simulink model "PubIfDecisionTOS_MDL"  (R2020b)
settings: configuration reference "DspaceConfig" (kept outside this file)
PostLoadFcn:
  | if any(exist('dsrtsu_mdlpostloadfcn', 'file') ~= 0), dsrtsu_mdlpostloadfcn('Execute', bdroot); end
InitFcn:
  | , if any(exist('dsmpb_private', 'file') ~= 0), dsmpb_private('dsmpb_mdlclblib', 'Init', bdroot); end,
undefined symbols (not defined in the file or in its folder): C_TOS_ACCEgoRAxletoFbumplength_m, C_TOS_ACCTargetFront_Flag, C_TOS_AEBJAPedObjDxThre_Val, C_TOS_AEBJAPedObjDyThre_Val, C_TOS_AEBJATargetSize_Val, C_TOS_AEBJAVehObjDxThre_Val, C_TOS_AEBJAVehObjDyThre_Val, C_TOS_AEBJuncPedTargetSize_Val, C_TOS_AEBLatObjDxThre_Val, C_TOS_AEBLatPedDyThre_Val, C_TOS_AEBLatTargetSize_Val, C_TOS_AEBLongTargetInEgoFront_Flag, C_TOS_axAbsGround_Parameter, C_TOS_CameraConfirmedFlag, C_TOS_CNsubjWidth, C_TOS_CurrentLaneCoreMinWidth_Val, C_TOS_CutInProb_Val_Zero, C_TOS_CutOutProb_Val_Zero, C_TOS_D2R_Val, C_TOS_DefaultValueObjectToCenterLine_dy, C_TOS_EgoCarWidth_Val, C_TOS_EgoDxRefPoint_m, C_TOS_EgoRAxletoFbumplength_m, C_TOS_HalfWidthVehicle_Con, C_TOS_HWA_CurrentLaneFlag, C_TOS_HWA_LeftLaneFlag, C_TOS_HWA_MovingDir_Vaild, C_TOS_HWA_MovState_Vaild, C_TOS_HWA_RightLaneFlag, C_TOS_LaneLineCourseErrorFront, C_TOS_LaneLineCourseErrorRear, C_TOS_MotorbikeDefaultWidth_m, C_TOS_NumberOfEffectiveTargets, C_TOS_Obj_Age_Val, C_TOS_Objdx_Constraint_Val, C_TOS_ObjectDefaultWidth_m, C_TOS_ObjInCurrentLane_Val, C_TOS_ObjInCurrentLaneValid, C_TOS_ObjInLeftLaneValid, C_TOS_ObjInRightLaneValid, C_TOS_ObjNotInCurrentLane_Val, C_TOS_ObjNotREElementType, C_TOS_ObjPredictDis_dy_ConstantVal_Zeros, C_TOS_ObjToCenterLine_ConstantVal_Zeros, C_TOS_OFMObjIDInvilad_Val, C_TOS_PIL_LatDisCons_Val_zero, C_TOS_PIL_ObjectCutInFlag_b, C_TOS_PIL_ObjectCutOutFlag_b, C_TOS_PIL_ObjLaneProb_al_Val, C_TOS_PP_ObjFusType_FC_Confirm_b, C_TOS_PP_ObjFusType_FC_FR_Confirm_b, C_TOS_PP_ObjFusType_FR_Confirm_b, C_TOS_RE_80BoolDefault_Val, C_TOS_RE_80Single181Default_Val, C_TOS_RE_80Single255Default_Val, C_TOS_RE_80Uint8Default_Val, C_TOS_RE_D2R, C_TOS_RE_D_180_Val, C_TOS_RE_InvalidObjectID_Val, C_TOS_RE_InvalidTargetChainDir_Val ... (+142)
libraries: simulink x1650, TOS_LIB x361, canfdmsglib x14
(part 62 of 69)

== stateflow chart PubIfDecisionTOS_MDL/TOS_20201112/TOS_2012080320/PIL_1029/OverlapRatio_Calculate/PIL_OverlapCalculation/OverlapRatioCalcFlow ==
  state overlapRatio = overlapRatioCalc(dyCriticalEgoObj,dyOverlapActual) [function]
  (default) -> (junction 33)
  (junction 33) -> (junction 2) : {
      | 	dyOverlapActual = dyEgo2Center - dyObject2Center;
      |
      | }
  (junction 2) -> (junction 3) [order 1] : [dyOverlapActual == 0]
  (junction 2) -> (junction 7) [order 2] : {
      | 	dyOverlapActualAbs = abs(dyOverlapActual);
      | }
  (junction 3) -> (junction 5) : {
      | 	tempOverlapRatio = 1;
      | }
  (junction 7) -> (junction 9) [order 1] : [dyOverlapActualAbs > dyCriticalEgoObj ]
  (junction 7) -> (junction 13) [order 2] : {
      | 	tempOverlapRatio = overlapRatioCalc(dyCriticalEgoObj,dyOverlapActual);
      | }
  (junction 9) -> (junction 11) : {
      | 	tempOverlapRatio = 0;
      | }
  (junction 11) -> (junction 13)
  (junction 5) -> (junction 11)
  (junction 13) -> (junction 17) : {
      | 	overlapRatio = tempOverlapRatio;
      | }
  data: dyCriticalEgoObj function_input; dyOverlapActual function_input; overlapRatio function_output; dyCriticalEgoObj input; dyEgo2Center input; overlapRatio output; tempOverlapRatio local double; dyOverlapActualAbs local double; dyObject2Center input; dyOverlapActual local double

== matlab function PubIfDecisionTOS_MDL/TOS_20201112/TOS_2012080320/PIL_1029/PIL_ObjectToCenterLine_dy_Filt/PIL_ObjectToCenterLine_dy/Subsystem/ObjectToCenterLine_dyFilit ==
  data: ObjectID_Filt_K1 input uint8; ObjectToCenterLine_dy_Filt_K1 input single; ObjectToCenterLine_dy input single; ObjectToCenterLine_dy_Filt output single; Object_ID input uint8; TOS_OFMObjValid_Flag input; P_TOS_PIL_ObjectToCenterLine_dy_CutInUpperLimit input single; P_TOS_PIL_ObjectToCenterLine_dy_CutInDeclineLimit input; Iterator_Num input int32
function ObjectToCenterLine_dy_Filt = fcn(ObjectID_Filt_K1,ObjectToCenterLine_dy_Filt_K1,ObjectToCenterLine_dy,...
    Object_ID,TOS_OFMObjValid_Flag,P_TOS_PIL_ObjectToCenterLine_dy_CutInUpperLimit,P_TOS_PIL_ObjectToCenterLine_dy_CutInDeclineLimit, Iterator_Num)

% Iterator_Num = uint8(80);
% K_FiltingParmet_RightLanepil=single(0);
ObjectToCenterLine_dy_Filt = single(0);


if  Object_ID ~=uint8(0) && TOS_OFMObjValid_Flag~=uint8(0)
        for  i=1: int32(Iterator_Num)
            if   ObjectID_Filt_K1(i) == Object_ID && ObjectID_Filt_K1(i)~=uint8(0)  && Object_ID~=uint8(0)   % 目标当前Object_ID 与历史值ObjectID_Filt_K1相同时；滤波处理

                    if ObjectToCenterLine_dy > ObjectToCenterLine_dy_Filt_K1(i) 
                          ObjectToCenterLine_dy_Filt = ObjectToCenterLine_dy_Filt_K1(i) + ...
                          P_TOS_PIL_ObjectToCenterLine_dy_CutInUpperLimit*( ObjectToCenterLine_dy - ObjectToCenterLine_dy_Filt_K1(i)); 
                    else
                         ObjectToCenterLine_dy_Filt = ObjectToCenterLine_dy_Filt_K1(i) + ...
                          P_TOS_PIL_ObjectToCenterLine_dy_CutInDeclineLimit*( ObjectToCenterLine_dy - ObjectToCenterLine_dy_Filt_K1(i)); 
                    end

                    break;
            else
                if i==Iterator_Num    % 如果当前Object_ID首次出现；输出当前值为ObjectToCenterLine_dy_Filt
                    ObjectToCenterLine_dy_Filt = ObjectToCenterLine_dy;        
                else
                    ObjectToCenterLine_dy_Filt = ObjectToCenterLine_dy;  
                end
            end 
        end
else
      ObjectToCenterLine_dy_Filt = ObjectToCenterLine_dy;  
end

== matlab function PubIfDecisionTOS_MDL/TOS_20201112/TOS_2012080320/PP1128/AAT-AdditionalAttributes/PP_ObjFirstDxDyDetermineSignalProcessing/PP_ObjFirstDxDyDetermine/PP_ObjFirstDxDyDetermine/MATLAB Function ==
  data: Object_ID input; Obj_DxFD output; Object_Dx input; Object_Dy input; Object_ID_Last input; Object_Dx_Last input; Object_Dy_Last input; Obj_DyFD output; C_NumberOfEffectiveTargets input
function [Obj_DxFD,Obj_DyFD] = fcn(Object_ID,Object_Dx,Object_Dy,Object_ID_Last,Object_Dx_Last,Object_Dy_Last,C_NumberOfEffectiveTargets)
objindex=uint8(0);
for i=1:C_NumberOfEffectiveTargets
    if Object_ID_Last(i)==Object_ID && Object_ID_Last(i)~=uint8(0)
        objindex=uint8(i);
        break
    end
end
if objindex~=0
    Obj_DxFD=single(Object_Dx_Last(objindex));
    Obj_DyFD=single(Object_Dy_Last(objindex));
else
    Obj_DxFD=single(Object_Dx);
    Obj_DyFD=single(Object_Dy);
end

== matlab function PubIfDecisionTOS_MDL/TOS_20201112/TOS_2012080320/PP1128/AAT-AdditionalAttributes/PP_ObjectToCenterLine_dy/PP_ObjectToCenterLine_vyc/ObjVyc ==
  data: ObjVyc output single; Line04_PC2 input single size=1; Line04_PC1 input single size=1; Line04_dDisStart input single size=1; Line04_dDisEnd input single size=1; Line05_PC2 input single size=1; Line05_PC1 input single size=1; Line05_dDisStart input single size=1; Line05_dDisEnd input single size=1; Line06_PC2 input single size=1; Line06_PC1 input single size=1; Line06_dDisStart input single size=1; Line06_dDisEnd input single size=1; Obj_ID input uint8 size=80; Obj_Dx input single size=80; Obj_VxG input single size=80; Obj_VyG input single size=80; TOS_OFMObjValid_Flag input uint8; vxvRefMs input; C_NumberOfEffectiveTargets input int32 size=1
function ObjVyc  = ObjVyc( Line04_PC2,Line04_PC1,Line04_dDisStart,Line04_dDisEnd,...
                           Line05_PC2,Line05_PC1,Line05_dDisStart,Line05_dDisEnd,...
                           Line06_PC2,Line06_PC1,Line06_dDisStart,Line06_dDisEnd,...
                           Obj_ID,Obj_Dx,Obj_VxG,Obj_VyG,TOS_OFMObjValid_Flag, vxvRefMs,C_NumberOfEffectiveTargets)

 Iterator_Num = int32(80);                      
                       
ObjVyc = single(zeros(Iterator_Num,1));

for i=int32(1):int32(C_NumberOfEffectiveTargets)
    if Obj_ID(i) ~= uint8(0) && TOS_OFMObjValid_Flag(i) ~= uint8(0)
       t_dxv = Obj_Dx(i);  %车体系X方向距离，目标到后轴中心距离
       t_VxG = vxvRefMs+Obj_VxG(i); %车体系目标X方向绝对速度
       t_VyG = Obj_VyG(i); %车体系y方向绝对速度（自车VY=0）
%---------------------------------------------------------------------------------------------------------------------     
       t_bParabolaYNLane = single(1);
       t_bParabolaXNLane = single(1);  
       
       if t_dxv > Line04_dDisStart && t_dxv < Line04_dDisEnd
           temp1 =  single(2)*Line04_PC2*t_dxv + Line04_PC1;
           t_bParabolaXNLane = -temp1;
       else
           if t_dxv > Line05_dDisStart && t_dxv < Line05_dDisEnd
                 temp1 =  single(2)*Line05_PC2*t_dxv + Line05_PC1;
                 t_bParabolaXNLane = -temp1;
           else
              if t_dxv > Line06_dDisStart && t_dxv < Line06_dDisEnd
                 temp1 =  single(2)*Line06_PC2*t_dxv + Line06_PC1;
                 t_bParabolaXNLane = -temp1; 
              end
           end           
       end
%-----------------------------------------------------------------------------------        
       t_bParabolaMag = mag(t_bParabolaXNLane,t_bParabolaYNLane); %t_bParabolaXNLane;一阶导数取反；；t_bParabolaYNLane=1
       
       t_bParabolaXNLane = t_bParabolaXNLane/t_bParabolaMag;  
       t_bParabolaYNLane = t_bParabolaYNLane/t_bParabolaMag;       
           temp1 = t_VxG*t_bParabolaXNLane;
           temp2 = t_VyG*t_bParabolaYNLane;      
       ObjVyc(i) = temp1 + temp2;
    else
       ObjVyc(i) = single(0);
    end
end
end

function out = mag(x,y) %向量模运算（k,1）
M = max(abs(x),abs(y));
N = min(abs(x),abs(y));
out = M + single(0.322)*N;   
end

== matlab function PubIfDecisionTOS_MDL/TOS_20201112/TOS_2012080320/PP1128/AAT-AdditionalAttributes/PP_ObjectToCenterLine_dy/PP_ObjectToCenterLine_vyc/PP_ObjectToCenterLine_vyc_Filt/ObjectToCenterLine_vyc/ObjectToCenterLine_vyc_Filt/ObjectToCenterLine_vyc_Filt ==
  data: ObjectID_Filt_K1 input uint8; ObjectToCenterLine_dy_Filt_K1 input single; ObjectToCenterLine_dy input single; ObjectToCenterLine_dy_Filt output single; Object_ID input uint8; TOS_OFMObjValid_Flag input; P_TOS_PIL_ObjectToCenterLine_dy_CutInUpperLimit input single; P_TOS_PIL_ObjectToCenterLine_dy_CutInDeclineLimit input; Iterator_Num input int32
function ObjectToCenterLine_dy_Filt = fcn(ObjectID_Filt_K1,ObjectToCenterLine_dy_Filt_K1,ObjectToCenterLine_dy,...
    Object_ID,TOS_OFMObjValid_Flag,P_TOS_PIL_ObjectToCenterLine_dy_CutInUpperLimit,P_TOS_PIL_ObjectToCenterLine_dy_CutInDeclineLimit, Iterator_Num)

% Iterator_Num = uint8(80);
% K_FiltingParmet_RightLanepil=single(0);
ObjectToCenterLine_dy_Filt = single(0);


if  Object_ID ~=uint8(0) && TOS_OFMObjValid_Flag~=uint8(0)
        for  i=1: int32(Iterator_Num)
            if   ObjectID_Filt_K1(i) == Object_ID && ObjectID_Filt_K1(i)~=uint8(0)  && Object_ID~=uint8(0)   % 目标当前Object_ID 与历史值ObjectID_Filt_K1相同时；滤波处理

                    if ObjectToCenterLine_dy > ObjectToCenterLine_dy_Filt_K1(i) 
                          ObjectToCenterLine_dy_Filt = ObjectToCenterLine_dy_Filt_K1(i) + ...
                          P_TOS_PIL_ObjectToCenterLine_dy_CutInUpperLimit*( ObjectToCenterLine_dy - ObjectToCenterLine_dy_Filt_K1(i)); 
                    else
                         ObjectToCenterLine_dy_Filt = ObjectToCenterLine_dy_Filt_K1(i) + ...
                          P_TOS_PIL_ObjectToCenterLine_dy_CutInDeclineLimit*( ObjectToCenterLine_dy - ObjectToCenterLine_dy_Filt_K1(i)); 
                    end

                    break;
            else
                if i==Iterator_Num    % 如果当前Object_ID首次出现；输出当前值为ObjectToCenterLine_dy_Filt
                    ObjectToCenterLine_dy_Filt = ObjectToCenterLine_dy;        
                else
                    ObjectToCenterLine_dy_Filt = ObjectToCenterLine_dy;  
                end
            end 
        end
else
      ObjectToCenterLine_dy_Filt = ObjectToCenterLine_dy;  
end

== stateflow chart PubIfDecisionTOS_MDL/TOS_20201112/TOS_2012080320/PP1128/AAT-AdditionalAttributes/RoadEdge/RE_2020_12_07/RoadEdge_V2/RoadEdgeElementFinalJudge/EgoLeft_RoadEdgeElementsFinalJudge/RoadEdgeElementFinalJudge ==
  state RoadEdgeElementInJudge [function]
    state RoadEdgeElementTheta1Cal [function]
      state StillTarget13_Theta = Theta_Cal(Target3_Dx,Target1_Dx,Target3_Dy,Target1_Dy,ObjectsSortIndex,ObjectsSortIndex_K1,RE_13TargetTheta_K1) [function]
      state [RE_TooNear2Target_Flag,P_RE_NearTargetThetaOffset] = TargetDisJudge(Target4_Dy,Target3_Dy,Target1_Dy,Target4_Dx,Target3_Dx,Target1_Dx) [function]
      (default) -> (junction 285) : {
          | OFM_Target1_Index = RE_StillObjectSortIndex[i-uint8(3)] - uint8(1) ;
          | OFM_Target3_Index = RE_StillObjectSortIndex[i-uint8(1)] - uint8(1) ;
          | OFM_Target4_Index = RE_StillObjectSortIndex[i] - uint8(1) ;
          | }
      (junction 285) -> (junction 286) : {
          | Target1_Dx = Object_Dx[OFM_Target1_Index] ;
          | Target3_Dx = Object_Dx[OFM_Target3_Index] ;
          | Target4_Dx = Object_Dx[OFM_Target4_Index] ;
          | Target1_Dy = Object_Dy[OFM_Target1_Index] ;
          | Target3_Dy = Object_Dy[OFM_Target3_Index] ;
          | Target4_Dy = Object_Dy[OFM_Target4_Index] ;
          | }
      (junction 286) -> (junction 287) : {
          | ObjectsSortIndex_K1 = RE_StillObjectSortIndex_K1[i];
          | ObjectsSortIndex = RE_StillObjectSortIndex[i];
          | RE_13TargetTheta_K1 = RE_13TargetTheta_ALL[i];
          |
          | StillTarget13_Theta = Theta_Cal(Target3_Dx,Target1_Dx,Target3_Dy,Target1_Dy,ObjectsSortIndex,ObjectsSortIndex_K1,RE_13TargetTheta_K1);
          | StillTarget13_Theta_ALL[i] = StillTarget13_Theta;
          | StillTarget34_13_Theta_ALL[i] = RE_2TargetTheta[i] - StillTarget13_Theta;
          |
          | }
      (junction 287) -> (junction 288) : {
          | [RE_TooNear2Target_Flag,P_RE_NearTargetThetaOffset] = TargetDisJudge(Target4_Dy,Target3_Dy,Target1_Dy,Target4_Dx,Target3_Dx,Target1_Dx);
          | RE_TooNear2Target_Flag_ALL[i] = RE_TooNear2Target_Flag;
          | }
      (junction 288) -> (junction 840)
    state RoadEdgeElement2ndInJudge [function]
      (default) -> (junction 249)
      (junction 249) -> (junction 250) [order 1] : [RE_3TargetTheta[i-uint8(1)] < P_TOS_RE_REE3TargetThetaMax_Val&&...
          | RE_3TargetTheta[i-uint8(1)] > P_TOS_RE_REE3TargetThetaMin_Val]
      (junction 249) -> (junction 257) [order 2] : {
          | RoadEdgeElementFlag[OFM_Target_Index] = false;
          | }
      (junction 250) -> (junction 251)
      (junction 251) -> (junction 252) [order 1] : [Ego_Vxv <= P_TOS_RE_RoadEdgeGroupEgoVxvThre_Val]
      (junction 251) -> (junction 255) [order 2]
      (junction 252) -> (junction 253)
      (junction 253) -> (junction 254) [order 1] : [RE_TooNear2Target_Flag_ALL[i] == false &&...
          | StillTarget34_13_Theta_ALL[i] < P_TOS_RE_LowSpeedREE4TargetThetaMax_Val&&...
          | StillTarget34_13_Theta_ALL[i] > P_TOS_RE_LowSpeedREE4TargetThetaMin_Val]
      (junction 253) -> (junction 854) [order 2]
      (junction 254) -> (junction 261) : {
          | RoadEdgeElementFlag[OFM_Target_Index] = true;
          | }
      (junction 255) -> (junction 256) [order 1] : [RE_TooNear2Target_Flag_ALL[i] == false &&...
          | StillTarget34_13_Theta_ALL[i] < P_TOS_RE_HighSpeedREE4TargetThetaMax_Val&&...
          | StillTarget34_13_Theta_ALL[i] > P_TOS_RE_HighSpeedREE4TargetThetaMin_Val]
      (junction 255) -> (junction 849) [order 2]
      (junction 256) -> (junction 259) : {
          | RoadEdgeElementFlag[OFM_Target_Index] = true;
          | }
      (junction 854) -> (junction 856) [order 1] : [RE_TooNear2Target_Flag_ALL[i] == true &&...
          | StillTarget34_13_Theta_ALL[i] < P_TOS_RE_LowSpeedREE4TargetThetaMax_Val + P_RE_NearTargetThetaOffset &&...
          | StillTarget34_13_Theta_ALL[i] > P_TOS_RE_LowSpeedREE4TargetThetaMin_Val - P_RE_NearTargetThetaOffset]
      (junction 854) -> (junction 260) [order 2] : {
          | RoadEdgeElementFlag[OFM_Target_Index] = false;
          | }
      (junction 856) -> (junction 858) : {
          | RoadEdgeElementFlag[OFM_Target_Index] = true;
          | }
      (junction 849) -> (junction 851) [order 1] : [RE_TooNear2Target_Flag_ALL[i] == true &&...
          | StillTarget34_13_Theta_ALL[i] < P_TOS_RE_HighSpeedREE4TargetThetaMax_Val + P_RE_NearTargetThetaOffset&&...
          | StillTarget34_13_Theta_ALL[i] > P_TOS_RE_HighSpeedREE4TargetThetaMin_Val - P_RE_NearTargetThetaOffset]
      (junction 849) -> (junction 258) [order 2] : {
          | RoadEdgeElementFlag[OFM_Target_Index] = false;
          | }
      (junction 851) -> (junction 846) : {
          | RoadEdgeElementFlag[OFM_Target_Index] = true;
          | }
      (junction 261) -> (junction 858)
      (junction 858) -> (junction 260)
      (junction 258) -> (junction 257)
      (junction 846) -> (junction 258)
      (junction 259) -> (junction 846)
      (junction 260) -> (junction 259)
      (junction 257) -> (junction 262)
    state RoadEdgeElement2ndOutJudge [function]
      (default) -> (junction 864)
      (junction 864) -> (junction 865) [order 1] : [RE_3TargetTheta[i-uint8(1)] < P_TOS_RE_REE3TargetThetaMax_Val&&...
          | RE_3TargetTheta[i-uint8(1)] > P_TOS_RE_REE3TargetThetaMin_Val]
      (junction 864) -> (junction 877) [order 2] : {
          | RoadEdgeElementFlag[OFM_Target_Index] = false;
          | }
      (junction 865) -> (junction 867)
      (junction 867) -> (junction 866) [order 1] : [Ego_Vxv <= P_TOS_RE_RoadEdgeGroupEgoVxvThre_Val]
      (junction 867) -> (junction 868) [order 2]
      (junction 866) -> (junction 873)
      (junction 873) -> (junction 874) [order 1] : [RE_TooNear2Target_Flag_ALL[i] == false &&...
          | StillTarget34_13_Theta_ALL[i] < P_TOS_RE_LowSpeedREE4TargetThetaMaxOut_Val&&...
          | StillTarget34_13_Theta_ALL[i] > P_TOS_RE_LowSpeedREE4TargetThetaMinOut_Val]
      (junction 873) -> (junction 903) [order 2]
      (junction 874) -> (junction 878) : {
          | RoadEdgeElementFlag[OFM_Target_Index] = true;
          | }
      (junction 868) -> (junction 872) [order 1] : [RE_TooNear2Target_Flag_ALL[i] == false &&...
          | StillTarget34_13_Theta_ALL[i] < P_TOS_RE_HighSpeedREE4TargetThetaMaxOut_Val&&...
          | StillTarget34_13_Theta_ALL[i] > P_TOS_RE_HighSpeedREE4TargetThetaMinOut_Val]
      (junction 868) -> (junction 898) [order 2]
      (junction 872) -> (junction 876) : {
          | RoadEdgeElementFlag[OFM_Target_Index] = true;
          | }
      (junction 903) -> (junction 863) [order 1] : [RE_TooNear2Target_Flag_ALL[i] == true &&...
          | StillTarget34_13_Theta_ALL[i] < P_TOS_RE_LowSpeedREE4TargetThetaMaxOut_Val + P_RE_NearTargetThetaOffset &&...
          | StillTarget34_13_Theta_ALL[i] > P_TOS_RE_LowSpeedREE4TargetThetaMinOut_Val - P_RE_NearTargetThetaOffset]
      (junction 903) -> (junction 871) [order 2] : {
          | RoadEdgeElementFlag[OFM_Target_Index] = false;
          | }
      (junction 863) -> (junction 861) : {
          | RoadEdgeElementFlag[OFM_Target_Index] = true;
          | }
      (junction 898) -> (junction 897) [order 1] : [RE_TooNear2Target_Flag_ALL[i] == true &&...
          | StillTarget34_13_Theta_ALL[i] < P_TOS_RE_HighSpeedREE4TargetThetaMaxOut_Val + P_RE_NearTargetThetaOffset&&...
          | StillTarget34_13_Theta_ALL[i] > P_TOS_RE_HighSpeedREE4TargetThetaMinOut_Val - P_RE_NearTargetThetaOffset]
      (junction 898) -> (junction 875) [order 2] : {
          | RoadEdgeElementFlag[OFM_Target_Index] = false;
          | }
      (junction 897) -> (junction 900) : {
          | RoadEdgeElementFlag[OFM_Target_Index] = true;
          | }
      (junction 878) -> (junction 861)
      (junction 861) -> (junction 871)
      (junction 875) -> (junction 877)
      (junction 900) -> (junction 875)
      (junction 876) -> (junction 900)
      (junction 871) -> (junction 876)
      (junction 877) -> (junction 869)
    state RoadEdgeElement3rdInJudge [function]
      (default) -> (junction 300)
      (junction 300) -> (junction 301) [order 1] : [RE_3TargetTheta[i-uint8(2)] < P_TOS_RE_REE3TargetThetaMax_Val&&...
          | RE_3TargetTheta[i-uint8(2)] > P_TOS_RE_REE3TargetThetaMin_Val]
      (junction 300) -> (junction 308) [order 2] : {
          | RoadEdgeElementFlag[OFM_Target_Index] = false;
          | }
      (junction 301) -> (junction 302)
      (junction 302) -> (junction 303) [order 1] : [Ego_Vxv <= P_TOS_RE_RoadEdgeGroupEgoVxvThre_Val]
      (junction 302) -> (junction 304) [order 2]
      (junction 303) -> (junction 306)
      (junction 306) -> (junction 307) [order 1] : [RE_TooNear2Target_Flag_ALL[i] == false &&...
          | (StillTarget34_13_Theta_ALL[i-uint8(1)] < P_TOS_RE_HighSpeedREE4TargetThetaMax_Val&&...
          | StillTarget34_13_Theta_ALL[i-uint8(1)] > P_TOS_RE_HighSpeedREE4TargetThetaMin_Val)&&...
          | (StillTarget34_13_Theta_ALL[i] < P_TOS_RE_LowSpeedREE4TargetThetaMax_Val&&...
          | StillTarget34_13_Theta_ALL[i] > P_TOS_RE_LowSpeedREE4TargetThetaMin_Val)]
      (junction 306) -> (junction 914) [order 2]
      (junction 307) -> (junction 312) : {
          | RoadEdgeElementFlag[OFM_Target_Index] = true;
          | }
      (junction 304) -> (junction 305) [order 1] : [RE_TooNear2Target_Flag_ALL[i] == false &&...
          | (StillTarget34_13_Theta_ALL[i-uint8(1)] < P_TOS_RE_HighSpeedREE4TargetThetaMax_Val&&...
          | StillTarget34_13_Theta_ALL[i-uint8(1)] > P_TOS_RE_HighSpeedREE4TargetThetaMin_Val)&&...
          | (StillTarget34_13_Theta_ALL[i] < P_TOS_RE_HighSpeedREE4TargetThetaMax_Val&&...
          | StillTarget34_13_Theta_ALL[i] > P_TOS_RE_HighSpeedREE4TargetThetaMin_Val)]
      (junction 304) -> (junction 907) [order 2]
      (junction 305) -> (junction 310) : {
          | RoadEdgeElementFlag[OFM_Target_Index] = true;
          | }
      (junction 914) -> (junction 916) [order 1] : [RE_TooNear2Target_Flag_ALL[i] == true &&...
          | (StillTarget34_13_Theta_ALL[i-uint8(1)] < P_TOS_RE_HighSpeedREE4TargetThetaMax_Val + P_RE_NearTargetThetaOffset&&...
          | StillTarget34_13_Theta_ALL[i-uint8(1)] > P_TOS_RE_HighSpeedREE4TargetThetaMin_Val - P_RE_NearTargetThetaOffset)&&...
          | (StillTarget34_13_Theta_ALL[i] < P_TOS_RE_LowSpeedREE4TargetThetaMax_Val + P_RE_NearTargetThetaOffset&&...
          | StillTarget34_13_Theta_ALL[i] > P_TOS_RE_LowSpeedREE4TargetThetaMin_Val - P_RE_NearTargetThetaOffset)]
      (junction 907) -> (junction 909) [order 1] : [RE_TooNear2Target_Flag_ALL[i] == true &&...
          | (StillTarget34_13_Theta_ALL[i-uint8(1)] < P_TOS_RE_HighSpeedREE4TargetThetaMax_Val + P_RE_NearTargetThetaOffset&&...
          | StillTarget34_13_Theta_ALL[i-uint8(1)] > P_TOS_RE_HighSpeedREE4TargetThetaMin_Val - P_RE_NearTargetThetaOffset)&&...
          | (StillTarget34_13_Theta_ALL[i] < P_TOS_RE_HighSpeedREE4TargetThetaMax_Val + P_RE_NearTargetThetaOffset&&...
          | StillTarget34_13_Theta_ALL[i] > P_TOS_RE_HighSpeedREE4TargetThetaMin_Val - P_RE_NearTargetThetaOffset)]
      (junction 914) -> (junction 311) [order 2] : {
          | RoadEdgeElementFlag[OFM_Target_Index] = false;
          | }
      (junction 916) -> (junction 918) : {
          | RoadEdgeElementFlag[OFM_Target_Index] = true;
          | }
      (junction 907) -> (junction 309) [order 2] : {
          | RoadEdgeElementFlag[OFM_Target_Index] = false;
          | }
      (junction 909) -> (junction 911) : {
          | RoadEdgeElementFlag[OFM_Target_Index] = true;
          | }
      (junction 309) -> (junction 308)
      (junction 911) -> (junction 309)
      (junction 310) -> (junction 911)
      (junction 311) -> (junction 310)
      (junction 918) -> (junction 311)
      (junction 312) -> (junction 918)
      (junction 308) -> (junction 313)
    state RoadEdgeElement3rdOutJudge [function]
      (default) -> (junction 924)
      (junction 924) -> (junction 921) [order 1] : [RE_3TargetTheta[i-uint8(2)] < P_TOS_RE_REE3TargetThetaMax_Val&&...
          | RE_3TargetTheta[i-uint8(2)] > P_TOS_RE_REE3TargetThetaMin_Val]
      (junction 924) -> (junction 934) [order 2] : {
          | RoadEdgeElementFlag[OFM_Target_Index] = false;
          | }
      (junction 921) -> (junction 933)
      (junction 933) -> (junction 927) [order 1] : [Ego_Vxv <= P_TOS_RE_RoadEdgeGroupEgoVxvThre_Val]
      (junction 933) -> (junction 925) [order 2]
      (junction 927) -> (junction 928)
      (junction 928) -> (junction 932) [order 1] : [RE_TooNear2Target_Flag_ALL[i] == false &&...
          | (StillTarget34_13_Theta_ALL[i-uint8(1)] < P_TOS_RE_HighSpeedREE4TargetThetaMaxOut_Val&&...
          | StillTarget34_13_Theta_ALL[i-uint8(1)] > P_TOS_RE_HighSpeedREE4TargetThetaMinOut_Val)&&...
          | (StillTarget34_13_Theta_ALL[i] < P_TOS_RE_LowSpeedREE4TargetThetaMaxOut_Val&&...
          | StillTarget34_13_Theta_ALL[i] > P_TOS_RE_LowSpeedREE4TargetThetaMinOut_Val)]
      (junction 928) -> (junction 965) [order 2]
      (junction 932) -> (junction 937) : {
          | RoadEdgeElementFlag[OFM_Target_Index] = true;
          | }
      (junction 925) -> (junction 938) [order 1] : [RE_TooNear2Target_Flag_ALL[i] == false &&...
          | (StillTarget34_13_Theta_ALL[i-uint8(1)] < P_TOS_RE_HighSpeedREE4TargetThetaMaxOut_Val&&...
          | StillTarget34_13_Theta_ALL[i-uint8(1)] > P_TOS_RE_HighSpeedREE4TargetThetaMinOut_Val)&&...
          | (StillTarget34_13_Theta_ALL[i] < P_TOS_RE_HighSpeedREE4TargetThetaMaxOut_Val&&...
          | StillTarget34_13_Theta_ALL[i] > P_TOS_RE_HighSpeedREE4TargetThetaMinOut_Val)]
      (junction 925) -> (junction 956) [order 2]
      (junction 938) -> (junction 929) : {
          | RoadEdgeElementFlag[OFM_Target_Index] = true;
          | }
      (junction 965) -> (junction 957) [order 1] : [RE_TooNear2Target_Flag_ALL[i] == true &&...
          | (StillTarget34_13_Theta_ALL[i-uint8(1)] < P_TOS_RE_HighSpeedREE4TargetThetaMaxOut_Val + P_RE_NearTargetThetaOffset&&...
          | StillTarget34_13_Theta_ALL[i-uint8(1)] > P_TOS_RE_HighSpeedREE4TargetThetaMinOut_Val - P_RE_NearTargetThetaOffset)&&...
          | (StillTarget34_13_Theta_ALL[i] < P_TOS_RE_LowSpeedREE4TargetThetaMaxOut_Val + P_RE_NearTargetThetaOffset&&...
          | StillTarget34_13_Theta_ALL[i] > P_TOS_RE_LowSpeedREE4TargetThetaMinOut_Val - P_RE_NearTargetThetaOffset)]
      (junction 956) -> (junction 962) [order 1] : [RE_TooNear2Target_Flag_ALL[i] == true &&...
          | (StillTarget34_13_Theta_ALL[i-uint8(1)] < P_TOS_RE_HighSpeedREE4TargetThetaMaxOut_Val + P_RE_NearTargetThetaOffset&&...
          | StillTarget34_13_Theta_ALL[i-uint8(1)] > P_TOS_RE_HighSpeedREE4TargetThetaMinOut_Val - P_RE_NearTargetThetaOffset)&&...
          | (StillTarget34_13_Theta_ALL[i] < P_TOS_RE_HighSpeedREE4TargetThetaMaxOut_Val + P_RE_NearTargetThetaOffset&&...
          | StillTarget34_13_Theta_ALL[i] > P_TOS_RE_HighSpeedREE4TargetThetaMinOut_Val - P_RE_NearTargetThetaOffset)]
      (junction 965) -> (junction 940) [order 2] : {
          | RoadEdgeElementFlag[OFM_Target_Index] = false;
          | }
      (junction 957) -> (junction 954) : {
          | RoadEdgeElementFlag[OFM_Target_Index] = true;
          | }
      (junction 956) -> (junction 936) [order 2] : {
          | RoadEdgeElementFlag[OFM_Target_Index] = false;
          | }
      (junction 962) -> (junction 959) : {
          | RoadEdgeElementFlag[OFM_Target_Index] = true;
          | }
      (junction 936) -> (junction 934)
      (junction 959) -> (junction 936)
      (junction 929) -> (junction 959)
      (junction 940) -> (junction 929)
      (junction 954) -> (junction 940)
      (junction 937) -> (junction 954)
      (junction 934) -> (junction 942)
    state RoadEdgeElement1stInJudge [function]
      (default) -> (junction 333)
      (junction 333) -> (junction 334) [order 1] : [RE_3TargetTheta[i] < P_TOS_RE_REE3TargetThetaMax_Val&&...
          | RE_3TargetTheta[i] > P_TOS_RE_REE3TargetThetaMin_Val]
      (junction 333) -> (junction 335) [order 2] : {
          | RoadEdgeElementFlag[OFM_Target_Index] = false;
          | }
      (junction 334) -> (junction 336) : {
          | RoadEdgeElementFlag[OFM_Target_Index_2 ] = true;
          | RoadEdgeElementFlag[OFM_Target_Index_1 ] = true;
          | RoadEdgeElementFlag[OFM_Target_Index] = true;
          | }
      (junction 336) -> (junction 335)
      (junction 335) -> (junction 337)
    (default) -> (junction 344) : {
        | OFM_Target_Index = RE_StillObjectSortIndex[i]-uint8(1) ;
        | OFM_Target_Index_1 = RE_StillObjectSortIndex[i-uint8(1)]-uint8(1) ;
        | OFM_Target_Index_2 = RE_StillObjectSortIndex[i-uint8(2)]-uint8(1) ;
        | }
    (junction 344) -> (junction 345) [order 1] : [EdgeGroupChainElementCount[i] == uint8(3)]
        | %一条边界组链中的第3个元素
    (junction 344) -> (junction 346) [order 2]
    (junction 345) -> (junction 360) : {
        | RoadEdgeElement1stInJudge();
        | }
    (junction 346) -> (junction 246) [order 1] : [EdgeGroupChainElementCount[i] >= uint8(4)]
        | %一条边界组链中的第4个和以后的元素
    (junction 346) -> (junction 282) [order 2] : {
        | RoadEdgeElementFlag[i] = false;
        | }
    (junction 246) -> (junction 281) : {
        | RoadEdgeElementTheta1Cal();
        | }
    (junction 281) -> (junction 247) [order 1] : [EdgeGroupChainElementCount[i] >= uint8(5)]
        | %一条边界组链中的第5个和以后的元素
    (junction 281) -> (junction 643) [order 2]
    (junction 247) -> (junction 636)
    (junction 636) -> (junction 638) [order 1] : [RE_4StepEdgeElementFlag[OFM_Target_Index] == true]
        | %连续四个周期选中为边界元素
    (junction 643) -> (junction 645) [order 1] : [RE_4StepEdgeElementFlag[OFM_Target_Index] == true]
        | %连续四个周期选中为边界元素
    (junction 636) -> (junction 362) [order 2] : {
        | RoadEdgeElement3rdInJudge();
        | }
    (junction 638) -> (junction 640) : {
        | RoadEdgeElement3rdOutJudge();
        | }
    (junction 643) -> (junction 283) [order 2] : {
        | RoadEdgeElement2ndInJudge();
        | }
    (junction 645) -> (junction 647) : {
        | RoadEdgeElement2ndOutJudge();
        | }
    (junction 283) -> (junction 282)
    (junction 647) -> (junction 283)
    (junction 362) -> (junction 647)
    (junction 640) -> (junction 362)
    (junction 360) -> (junction 640)
    (junction 282) -> (junction 480)
  state RoadEdgeElementOFMSort [function]
    (default) -> (junction 489)
    (junction 489) -> (junction 506) [order 1] : [RoadEdgeElementFlag[OFM_Target_Index] == true]
    (junction 489) -> (junction 495) [order 2] : %donothing
    (junction 506) -> (junction 502) : {
        | RE_EdgeElementType[OFM_Target_Index] = uint8(1);
        | RE_EdgeElementID[OFM_Target_Index] = Object_ID[OFM_Target_Index];
        | }
    (junction 502) -> (junction 494) [order 1] : [RoadEdgeElementFlag[OFM_Target_Index_1] == true]
    (junction 502) -> (junction 505) [order 2] : %donothing
    (junction 494) -> (junction 504) : {
        | RE_EdgeElementType[OFM_Target_Index_1] = uint8(1);
        | RE_EdgeElementID[OFM_Target_Index_1] = Object_ID[OFM_Target_Index_1];
        | }
    (junction 504) -> (junction 499) [order 1] : [RoadEdgeElementFlag[OFM_Target_Index_2] == true]
    (junction 504) -> (junction 492) [order 2] : %donothing
    (junction 499) -> (junction 493) : {
        | RE_EdgeElementType[OFM_Target_Index_2] = uint8(1);
        | RE_EdgeElementID[OFM_Target_Index_2] = Object_ID[OFM_Target_Index_2];
        | }
    (junction 505) -> (junction 495)
    (junction 492) -> (junction 505)
    (junction 493) -> (junction 492)
    (junction 495) -> (junction 512)
  state RoadEdgeElementInfo_OFM [function]
    (default) -> (junction 982) : {
        | OFM_Target_Index = RE_StillObjectSortIndex[i]-uint8(1) ;
        | }
    (junction 982) -> (junction 983) : {
        | EdgeGroupChainElementCount_OFM[OFM_Target_Index] = EdgeGroupChainElementCount[i];
        | EdgeGroupChainElementCount_OFM[RE_StillObjectSortIndex[0]-uint8(1)] = EdgeGroupChainElementCount[0];
        | EdgeGroupChainElementCount_OFM[RE_StillObjectSortIndex[1]-uint8(1)] = EdgeGroupChainElementCount[1];
        |
        | StillTarget13_Theta_OFM[OFM_Target_Index] = StillTarget13_Theta;
        | StillTarget34_13_Theta_OFM[OFM_Target_Index] = StillTarget34_13_Theta_ALL[i];
        | StillTarget3Theta_OFM[OFM_Target_Index] = RE_3TargetTheta[i];
        | StillTarget2Theta_OFM[OFM_Target_Index] = RE_2TargetTheta[i];
        |
        |
        | StillTarget2Theta_OFM[RE_StillObjectSortIndex[0]-uint8(1)] = RE_2TargetTheta[0];
        |
        |
        | StillTarget3Theta_OFM[RE_StillObjectSortIndex[1]-uint8(1)] = RE_3TargetTheta[1];
        | StillTarget2Theta_OFM[RE_StillObjectSortIndex[1]-uint8(1)] = RE_2TargetTheta[1];
        | }
    (junction 983) -> (junction 1006)
  (default) -> (junction 35) : {
      | i = uint8(2);
      | RoadEdgeElementFlag = C_TOS_RE_80BoolDefault_Val;
      | RE_EdgeElementType = C_TOS_RE_80Uint8Default_Val;
      | RE_EdgeElementID = C_TOS_RE_80Uint8Default_Val;
      | StillTarget13_Theta = single(181);
      | StillTarget34_13_Theta_ALL = C_TOS_RE_80Single181Default_Val;
      | EdgeGroupChainElementCount_OFM = C_TOS_RE_80Uint8Default_Val;
      |
      | StillTarget2Theta_OFM = C_TOS_RE_80Single181Default_Val;
      | StillTarget3Theta_OFM = C_TOS_RE_80Single181Default_Val;
      | StillTarget34_13_Theta_OFM = C_TOS_RE_80Single181Default_Val;
      | StillTarget13_Theta_OFM = C_TOS_RE_80Single181Default_Val;%观测量
      | }
      | %从第三个目标开始计算判断
  (junction 35) -> (junction 37) [order 1] : [RE_StillObjectSortIndex[i] ~= C_TOS_StillObjSortInvalidIndex_Val &&...
      | i <= uint8(79)]
  (junction 978) -> (junction 35) : {
      | i = i+uint8(1);
      | }
  (junction 35) -> (junction 40) [order 2]
  (junction 37) -> (junction 514) : {
      | RoadEdgeElementInJudge();
      | }
  (junction 514) -> (junction 515) : {
      | RoadEdgeElementOFMSort();
      | }
  (junction 40) -> (junction 43)
  (junction 515) -> (junction 978) : {
      | RoadEdgeElementInfo_OFM();
      | }
  data: Target3_Dx function_input single size=1; Target1_Dx function_input single size=1; Target3_Dy function_input single size=1; Target1_Dy function_input single size=1; StillTarget13_Theta function_output single size=1; ObjectsSortIndex function_input; ObjectsSortIndex_K1 function_input; RE_13TargetTheta_K1 function_input; Target4_Dy function_input single size=1; Target3_Dy function_input single size=1; Target1_Dy function_input single size=1; Target4_Dx function_input single size=1; Target3_Dx function_input single size=1; Target1_Dx function_input single size=1; RE_TooNear2Target_Flag function_output; P_RE_NearTargetThetaOffset function_output; RE_4StepEdgeElementFlag input; C_TOS_StillObjSortInvalidIndex_Val parameter; EdgeGroupChainElementCount input; RE_3TargetTheta input; RE_2TargetTheta input; RE_StillObjectSortIndex input; RE_StillObjectSortIndex_K1 input; Ego_Vxv input; Object_Dx input; Object_Dy input; P_TOS_RE_REE3TargetThetaMax_Val parameter; P_TOS_RE_REE3TargetThetaMin_Val parameter; P_TOS_RE_HighSpeedREE4TargetThetaMax_Val parameter; P_TOS_RE_HighSpeedREE4TargetThetaMin_Val parameter; P_TOS_RE_LowSpeedREE4TargetThetaMax_Val parameter; P_TOS_RE_LowSpeedREE4TargetThetaMin_Val parameter; P_TOS_RE_RoadEdgeGroupEgoVxvThre_Val parameter; OFM_Target1_Index local uint8 size=1; OFM_Target3_Index local uint8 size=1; Target1_Dx local single size=1; Target1_Dy local single size=1; Target3_Dx local single size=1; Target3_Dy local single size=1; i local uint8 size=1; RoadEdgeElementFlag output boolean size=80; Object_ID input; RE_EdgeElementType output uint8 size=80; OFM_Target_Index local uint8 size=1; C_TOS_RE_80BoolDefault_Val parameter; C_TOS_RE_80Single181Default_Val parameter; C_TOS_RE_80Uint8Default_Val parameter; StillTarget34_13_Theta_ALL output single size=80; StillTarget13_Theta local single size=1; RE_EdgeElementID output uint8 size=80; P_TOS_RE_HighSpeedREE4TargetThetaMaxOut_Val parameter; P_TOS_RE_HighSpeedREE4TargetThetaMinOut_Val parameter; P_TOS_RE_LowSpeedREE4TargetThetaMaxOut_Val parameter; P_TOS_RE_LowSpeedREE4TargetThetaMinOut_Val parameter; OFM_Target_Index_1 local uint8; OFM_Target_Index_2 local uint8; RE_13TargetTheta_ALL input; StillTarget13_Theta_ALL output single size=80; ObjectsSortIndex local uint8; ObjectsSortIndex_K1 local uint8; RE_13TargetTheta_K1 local single; StillTarget13_Theta_OFM output single size=80; StillTarget34_13_Theta_OFM output single size=80; StillTarget3Theta_OFM output single size=80; StillTarget2Theta_OFM output single size=80; EdgeGroupChainElementCount_OFM output uint8 size=80; P_RE_NearTargetThetaOffset local single; OFM_Target4_Index local uint8 size=1; RE_TooNear2Target_Flag local boolean size=1; RE_TooNear2Target_Flag_ALL local boolean size=80; Target4_Dx local single size=1; Target4_Dy local single size=1
